simulink model "stellaris_test_adc"  (R2013a)
settings: Solver=FixedStepDiscrete  StartTime=0.0  StopTime=10.0  FixedStep=0.01  RelTol=1e-3
undefined symbols (not defined in the file or in its folder): ADC_CTL_TS, ADC_TRIGGER_ALWAYS, ADC_TRIGGER_PROCESSOR, ADC_TRIGGER_TIMER, None
libraries: stellaris_lib x2
settings Model: Creator=peselnikmg  LastModifiedBy=peselnikmg
settings DataIOCC: SignalLoggingSaveFormat=ModelDataLogs
settings OptimizationCC: OptimizeModelRefInitCode=on  LifeSpan=1
settings HardwareCC: ProdEndianess=LittleEndian  ProdHWDeviceType=Texas Instruments->TMS470
settings RTWCC: SystemTargetFile=stellaris.tlc  TemplateMakefile=stellaris_tmf  PostCodeGenCommand=stellaris_customcode(buildInfo)  Description=TI Stellaris LaunchPad  ProcessScript=stellaris_make_rtw_hook
settings CodeAppCC: IgnoreCustomStorageClasses=off
settings STFCustomTargetCC: CombineOutputUpdateFcns=on  ERTCustomFileBanners=on  SupportContinuousTime=off  SupportNonInlinedSFcns=off  MATLABClassNameForMDSCustomization=Simulink.SoftwareTarget.ERTCustomization  SystemTargetFile=stellaris.tlc
settings ERTTargetCC: GenerateSampleERTMain=off  ParMdlRefBuildCompliant=off  CompOptLevelCompliant=off  ConcurrentExecutionCompliant=off  ERTFirstTimeCompliant=off  ModelStepFunctionPrototypeControlCompliant=off  CPPClassGenCompliant=off  ERTCustomFileTemplate=stellaris_srmain.tlc

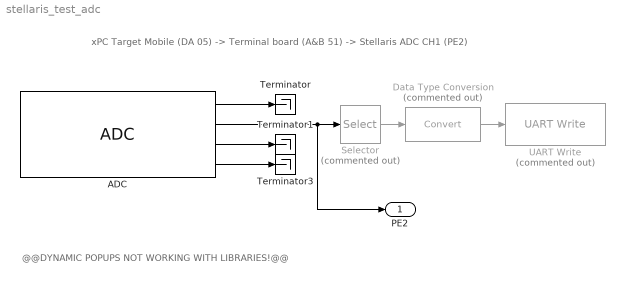
== system stellaris_test_adc ==
  note: @@DYNAMIC POPUPS NOT WORKING WITH LIBRARIES!@@
  note: xPC Target Mobile (DA 05) -> Terminal board (A&B 51) -> Stellaris ADC CH1 (PE2)
  ADC : stellaris_lib/ADC/ADC  ulBase=ADC0  ulFactor=64  SS0_ENA=disable  ulTrigger_SS0=ADC_TRIGGER_PROCESSOR(0)  ulPriority_SS0=0  ulConfig_SS0_1=----  Config_SS0_1=None(0)  ulConfig_SS0_2=----  Config_SS0_2=None(0)  ulConfig_SS0_3=----  Config_SS0_3=None(0)  ulConfig_SS0_4=----  Config_SS0_4=None(0)  ulConfig_SS0_5=----  Config_SS0_5=None(0)  ulConfig_SS0_6=----  Config_SS0_6=None(0)  ulConfig_SS0_7=----  Config_SS0_7=None(0)  ulConfig_SS0_8=----  Config_SS0_8=None(0)  SS1_ENA=enable  ulTrigger_SS1=ADC_TRIGGER_PROCESSOR(0)  ulPriority_SS1=1  ulConfig_SS1_1=----  Config_SS1_1=ADC_CTL_TS(128)  ulConfig_SS1_2=----  Config_SS1_2=ADC_CTL_TS(128)  ulConfig_SS1_3=----  Config_SS1_3=ADC_CTL_TS(128)  ulConfig_SS1_4=----  Config_SS1_4=ADC_CTL_TS|ADC_CTL_IE|ADC_CTL_END(224)  SS2_ENA=disable  ulTrigger_SS2=ADC_TRIGGER_TIMER(5)  ulPriority_SS2=2  ulConfig_SS2_1=----  Config_SS2_1=None(0)  ulConfig_SS2_2=----  Config_SS2_2=None(0)  ulConfig_SS2_3=----  Config_SS2_3=None(0)  ulConfig_SS2_4=----  Config_SS2_4=None(0)  SS3_ENA=disable  ulTrigger_SS3=ADC_TRIGGER_ALWAYS(15)  ulPriority_SS3=3  ulConfig_SS3_1=----  Config_SS3_1=None(0)  ulSpeed=SYSCTL_ADCSPEED_250KSPS
  Data Type Conversion : DataTypeConversion  Commented=on
  Selector : Selector  Commented=on  IndexMode=Zero-based  InputPortWidth=4  IndexOptions=Index vector (dialog)  Indices=[0]  OutputSizes=1
  Terminator : Terminator
  Terminator1 : Terminator
  Terminator3 : Terminator
  UART Write : stellaris_lib/UART/UART Write  Commented=on  nbFlag=on
  PE2 : Outport
  wires:
  ADC/2 -> PE2/1, Selector/1
  ADC/1 -> Terminator/1
  ADC/3 -> Terminator1/1
  ADC/4 -> Terminator3/1
  Selector/1 -> Data Type Conversion/1
  Data Type Conversion/1 -> UART Write/1
